simulink model "joy_stick_waypoints"  (R2024b)
settings: Solver=FixedStepAuto  StartTime=0.0  StopTime=inf  FixedStep=0.01  RelTol=1e-3
libraries: vrlib x3, aerolibutil x2
settings Model: Creator=vince  LastModifiedBy=vince

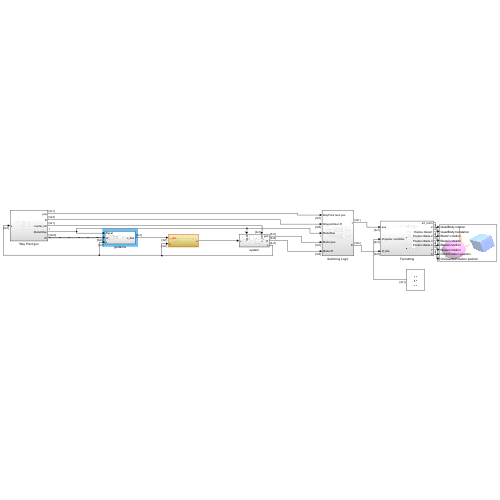
[thumbnail: Simulink's stored preview of the top-level diagram]
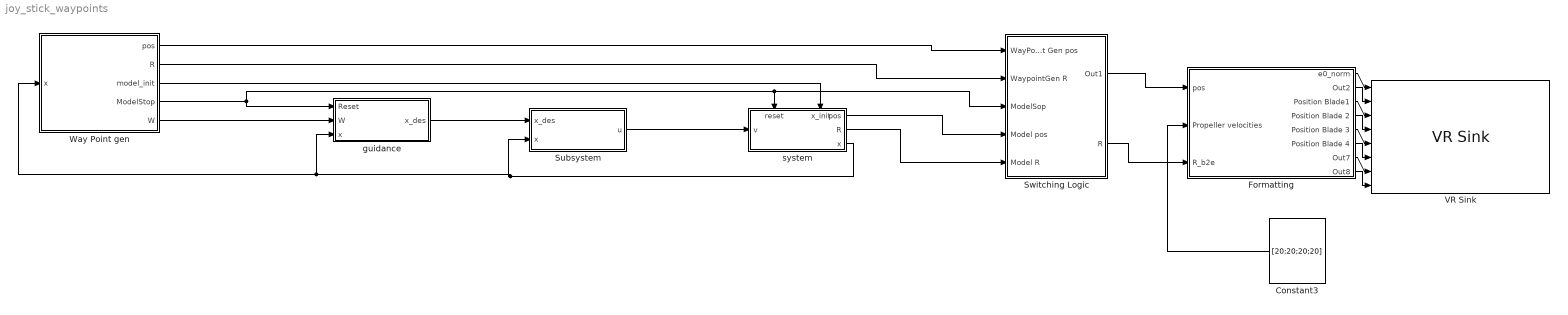
== system joy_stick_waypoints ==
  Constant3 : Constant  Value=[20;20;20;20]  VectorParams1D=off
  Formatting : Subsystem
  Subsystem : Subsystem
  Switching Logic : Subsystem
  VR Sink : vrlib/VR Sink  InstantiateOnLoad=on  SampleTime=12*0.005  ViewEnable=on  RemoteChange=off  RemoteView=off  FieldsWritten=QuadBody.rotation.4.1.1.double#QuadBody.translation.3.1.1.double#Blade1.rotation.4.1.1.double#Blade3.rotation.4.1.1.double#Blade2.rotation.4.1.1.double#Blade4.rotation.4.1.1.double#IsoNoRotation.position.3.1.1.double#OnQuadNoRotation.position.3.1.1.double  WorldFileName=Quadcopter_VR.wrl  AutoView=on  VideoDimensions=[]  AllowVariableSize=off  FigureProperties="{'Position', 'Name', 'Viewpoint', 'CameraBound', 'CameraDirection', 'CameraPosition', 'CameraUpVector', 'ZoomFactor', 'Antialiasing', 'Headlight', 'Lighting', 'Sound', 'StatusBar', 'Stereo3D', 'Stereo3DCameraOffset', 'Stereo3DHIT', 'ToolBar', 'Textures', 'Transparency', 'Triad', 'Wireframe', 'NavZones', 'NavMode', 'NavSpeed', 'CaptureFileFormat', 'CaptureFileName', 'Record2DCompressMethod', 'Record2DCompressQuality', 'Record2D', 'Record2DFileName', 'Record2DFPS', 'NavPanel'; [1.8747142857142856e+03   6.0128571428571422e+02   5.7600000000000000e+02   3.5000000000000000e+02], '', 'Chase - No Rotation', 'on', [0.0000000000000000e+00   0.0000000000000000e+00  -1.0000000000000000e+00], [0.0000000000000000e+00   0.0000000000000000e+00   0.0000000000000000e+00], [0.0000000000000000e+00   1.0000000000000000e+00   0.0000000000000000e+00], [1.0000000000000000e+00], 'on', 'on', 'on', 'on', 'on', 'off', [1.0000000149011612e-01], [0.0000000000000000e+00], 'on', 'on', 'on', 'none', 'off', 'off', 'fly', 'normal', 'tif', '%f_anim_%n.tif', 'auto', [7.5000000000000000e+01], 'off', '%f_anim_%n.avi', 'auto', 'halfbar'}"
  Way Point gen : Subsystem
  guidance : Subsystem
  system : Subsystem
      settings: PortSchema="{\"entries\":[{\"content\":{\"sides\":[{\"content\":{\"connectorIds\":[\"In1\"]},\"type\":\"ConnectorPlacement.EquallySpacedRectSide\",\"uuid\":\"24ab920f-ecdf-46b8-bd8f-9678a712bec3\"},{\"content\":{\"connectorIds\":[\"Out1\",\"Out2\",\"Out3\"],\"side\":\"RIGHT\"},\"type\":\"ConnectorPlacement.EquallySpacedRectSide\",\"uuid\":\"385c249c-ba59-490a-8b19-b03d9723e494\"},{\"content\":{\"connectorIds\":[\"In2\",\"In3\"],\"side\":\"TOP\"},\"type\":\"ConnectorPlacement.EquallySpacedRectSide\",\"uuid\":\"86d78a8a-2549-4abc-bd3a-7c80a79ae3d5\"}]},\"type\":\"ConnectorPlacement.EquallySpacedConnector\",\"uuid\":\"734c9ef5-af39-4002-a137-da897c88a198\"}],\"packageUris\":[\"http://schema.mathworks.com/mf0/Connector/R2020b\"],\"version\":\"1.0\"}"
  wires:
  Constant3/1 -> Formatting/2(Propeller velocities)
  Formatting/4(Position Blade 2) -> VR Sink/4
  Formatting/1(e0_norm) -> VR Sink/1
  Formatting/3(Position Blade1) -> VR Sink/3
  Formatting/8(Out8) -> VR Sink/8
  Formatting/7(Out7) -> VR Sink/7
  Formatting/5(Position Blade 3) -> VR Sink/5
  Formatting/6(Position Blade 4) -> VR Sink/6
  Formatting/2(Out2) -> VR Sink/2
  system/1(pos) -> Switching Logic/4(Model pos)
  Subsystem/1(u) -> system/1(v)
  guidance/1(x_des) -> Subsystem/1(x_des)
  Way Point gen/5(W) -> guidance/2(W)
  Way Point gen/3(model_init) -> system/3(x_init)
  Way Point gen/1(pos) -> Switching Logic/1(WayPoint Gen pos)
  Switching Logic/1(Out1) -> Formatting/1(pos)
  Switching Logic/2(R) -> Formatting/3(R_b2e)
  system/2(R) -> Switching Logic/5(Model R)
  system/3(x) -> Way Point gen/1(x), guidance/3(x), Subsystem/2(x)
  Way Point gen/4(ModelStop) -> system/2(reset), Switching Logic/3(ModelSop), guidance/1(Reset)
  Way Point gen/2(R) -> Switching Logic/2(WaypointGen R)

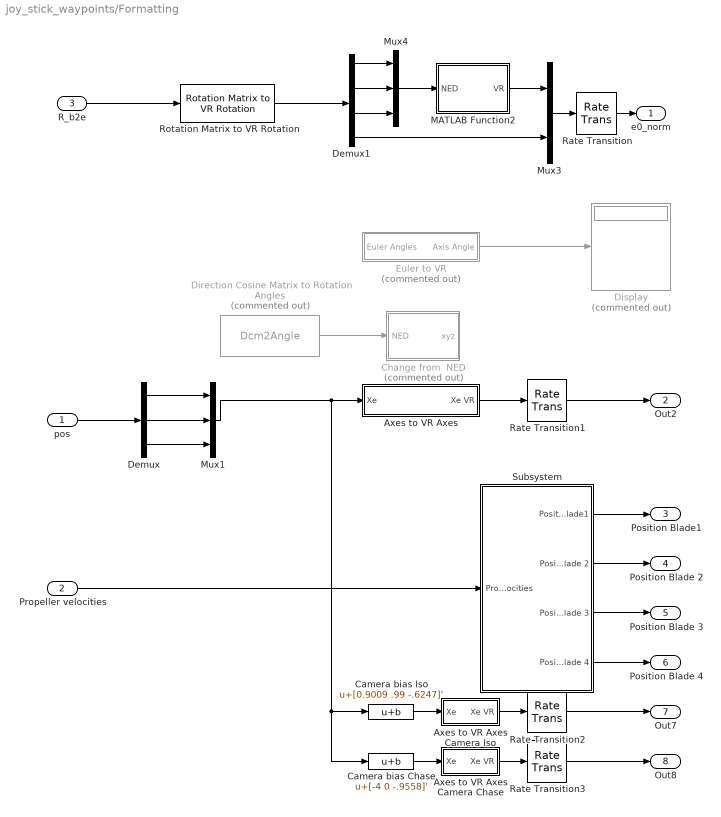
== system joy_stick_waypoints/Formatting ==
  pos : Inport
  Propeller velocities : Inport  Port=2
  R_b2e : Inport  Port=3
  Axes to VR Axes : Subsystem
  Axes to VR Axes Camera Chase : Subsystem
  Axes to VR Axes Camera Iso : Subsystem
  Camera bias Chase : Bias  Bias=[-4 0 -.9558]'  SaturateOnIntegerOverflow=off
  Camera bias Iso : Bias  Bias=[0.9009 .99 -.6247]'  SaturateOnIntegerOverflow=off
  Change from  NED : MATLAB Function  Commented=on  TreatAsAtomicUnit=on
  Demux : Demux  Outputs=3
  Demux1 : Demux
  Direction Cosine Matrix to Rotation Angles : Dcm2Angle  Commented=on
      settings: AttributesFormatString=Rotation Order: %<rotationOrder>
  Display : Display  Commented=on
  Euler to VR : Subsystem  Commented=on
  MATLAB Function2 : MATLAB Function  TreatAsAtomicUnit=on
  Mux1 : Mux  Inputs=3
  Mux3 : Mux  Inputs=2
  Mux4 : Mux  Inputs=3
  Rate Transition{,1..3} (4 alike) : RateTransition
  Rotation Matrix to VR Rotation : vrlib/Utilities/Rotation Matrix to VR Rotation  maxzero=1e-12
  Subsystem : Subsystem
  e0_norm : Outport
  Out2 : Outport  Port=2
  Position Blade1 : Outport  Port=3
  Position Blade 2 : Outport  Port=4
  Position Blade 3 : Outport  Port=5
  Position Blade 4 : Outport  Port=6
  Out7 : Outport  Port=7
  Out8 : Outport  Port=8
  wires:
  Rate Transition2/1 -> Out7/1
  Propeller velocities/1 -> Subsystem/1(Propeller velocities)
  Subsystem/3(Position Blade 3) -> Position Blade 3/1
  Subsystem/1(Position Blade1) -> Position Blade1/1
  Camera bias Chase/1 -> Axes to VR Axes Camera Chase/1(Xe)
  Axes to VR Axes Camera Chase/1(Xe VR) -> Rate Transition3/1
  Subsystem/2(Position Blade 2) -> Position Blade 2/1
  Axes to VR Axes Camera Iso/1(Xe VR) -> Rate Transition2/1
  Axes to VR Axes/1(Xe VR) -> Rate Transition1/1
  Rate Transition1/1 -> Out2/1
  Camera bias Iso/1 -> Axes to VR Axes Camera Iso/1(Xe)
  Mux1/1 -> Camera bias Chase/1, Camera bias Iso/1, Axes to VR Axes/1(Xe)
  Rate Transition3/1 -> Out8/1
  Subsystem/4(Position Blade 4) -> Position Blade 4/1
  Demux/2 -> Mux1/2
  Demux/3 -> Mux1/3
  pos/1 -> Demux/1
  Demux/1 -> Mux1/1
  Euler to VR/1(Axis Angle) -> Display/1
  Direction Cosine Matrix to Rotation Angles/1 -> Change from  NED/1(NED)
  Demux1/1 -> Mux4/1
  Demux1/2 -> Mux4/2
  MATLAB Function2/1(VR) -> Mux3/1
  R_b2e/1 -> Rotation Matrix to VR Rotation/1
  Mux4/1 -> MATLAB Function2/1(NED)
  Rotation Matrix to VR Rotation/1 -> Demux1/1
  Demux1/4 -> Mux3/2
  Demux1/3 -> Mux4/3
  Mux3/1 -> Rate Transition/1
  Rate Transition/1 -> e0_norm/1

== system joy_stick_waypoints/Subsystem ==
  x_des : Inport
  x : Inport  Port=2
  Gain : Gain  Gain=-eye(4)  Multiplication=Matrix(K*u)
  Sum : Sum  Inputs=|-+
  u : Outport
  wires:
  Gain/1 -> u/1
  Sum/1 -> Gain/1
  x/1 -> Sum/2
  x_des/1 -> Sum/1

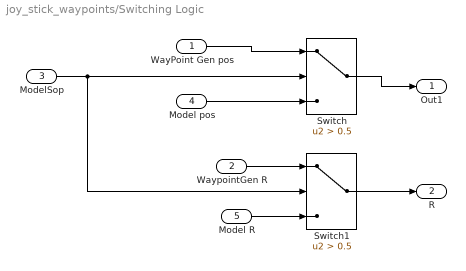
== system joy_stick_waypoints/Switching Logic ==
  WayPoint Gen pos : Inport
  WaypointGen R : Inport  Port=2
  ModelSop : Inport  Port=3
  Model pos : Inport  Port=4
  Model R : Inport  Port=5
  Switch : Switch  Criteria=u2 > Threshold  Threshold=0.5  SaturateOnIntegerOverflow=off  InputSameDT=off
  Switch1 : Switch  Criteria=u2 > Threshold  Threshold=0.5  SaturateOnIntegerOverflow=off  InputSameDT=off
  Out1 : Outport
  R : Outport  Port=2
  wires:
  Model pos/1 -> Switch/3
  ModelSop/1 -> Switch1/2, Switch/2
  WayPoint Gen pos/1 -> Switch/1
  Switch/1 -> Out1/1
  WaypointGen R/1 -> Switch1/1
  Model R/1 -> Switch1/3
  Switch1/1 -> R/1

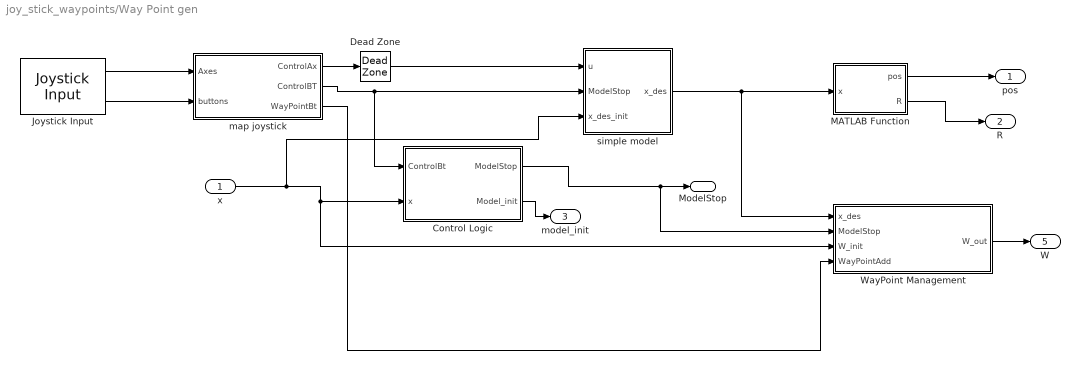
== system joy_stick_waypoints/Way Point gen ==
  x : Inport
  Control Logic : Subsystem
  Dead Zone : DeadZone  LowerValue=-0.1  UpperValue=0.1
  Joystick Input : vrlib/Joystick Input  joyid=1  adjustports=on  forcefeed=off
  MATLAB Function : MATLAB Function  TreatAsAtomicUnit=on
  WayPoint Management : MATLAB Function  TreatAsAtomicUnit=on
  map joystick : MATLAB Function  TreatAsAtomicUnit=on
  simple model : Subsystem
  pos : Outport
  R : Outport  Port=2
  model_init : Outport  Port=3
  ModelStop : Outport  Port=4
  W : Outport  Port=5
  wires:
  Joystick Input/2 -> map joystick/2(buttons)
  Joystick Input/1 -> map joystick/1(Axes)
  map joystick/1(ControlAx) -> Dead Zone/1
  Dead Zone/1 -> simple model/1(u)
  map joystick/2(ControlBT) -> Control Logic/1(ControlBt), simple model/2(ModelStop)
  x/1 -> WayPoint Management/3(W_init), Control Logic/2(x), simple model/3(x_des_init)
  simple model/1(x_des) -> MATLAB Function/1(x), WayPoint Management/1(x_des)
  map joystick/3(WayPointBt) -> WayPoint Management/4(WayPointAdd)
  WayPoint Management/1(W_out) -> W/1
  Control Logic/1(ModelStop) -> ModelStop/1, WayPoint Management/2(ModelStop)
  Control Logic/2(Model_init) -> model_init/1
  MATLAB Function/1(pos) -> pos/1
  MATLAB Function/2(R) -> R/1

== system joy_stick_waypoints/guidance ==
  Reset : Inport
  W : Inport  Port=2
  x : Inport  Port=3
  select way point : MATLAB Function  TreatAsAtomicUnit=on
  x_des : Outport
  wires:
  W/1 -> select way point/1(W)
  x/1 -> select way point/2(x)
  select way point/1(x_des) -> x_des/1
  Reset/1 -> select way point/3(reset)

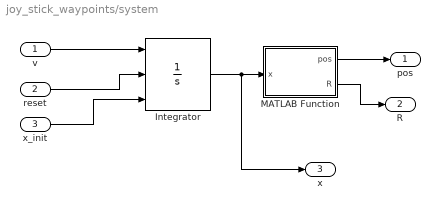
== system joy_stick_waypoints/system ==
  v : Inport
  reset : Inport  Port=2
  x_init : Inport  Port=3
  Integrator : Integrator  Priority=1  ExternalReset=level  InitialConditionSource=external
  MATLAB Function : MATLAB Function  TreatAsAtomicUnit=on
  pos : Outport
  R : Outport  Port=2
  x : Outport  Port=3
  wires:
  v/1 -> Integrator/1
  x_init/1 -> Integrator/3
  reset/1 -> Integrator/2
  MATLAB Function/1(pos) -> pos/1
  MATLAB Function/2(R) -> R/1
  Integrator/1 -> x/1, MATLAB Function/1(x)

== system joy_stick_waypoints/Formatting/Axes to VR Axes ==
  Xe : Inport
  Demux : Demux  Outputs=3
      settings: DisplayOption=none
  Mux : Mux  Inputs=3
  rad-->deg1 : Gain  Gain=-1  SaturateOnIntegerOverflow=on  OutDataTypeStr=Inherit: Same as input  ParamDataTypeStr=Inherit: Same as input
  Xe VR : Outport  VectorParamsAs1DForOutWhenUnconnected=off
  wires:
  Xe/1 -> Demux/1
  Demux/1 -> Mux/1
  Demux/3 -> rad-->deg1/1
  Mux/1 -> Xe VR/1
  rad-->deg1/1 -> Mux/2
  Demux/2 -> Mux/3

== system joy_stick_waypoints/Formatting/Axes to VR Axes Camera Chase ==
  Xe : Inport
  Demux : Demux  Outputs=3
      settings: DisplayOption=none
  Mux : Mux  Inputs=3
  rad-->deg1 : Gain  Gain=-1  SaturateOnIntegerOverflow=on  OutDataTypeStr=Inherit: Same as input  ParamDataTypeStr=Inherit: Same as input
  Xe VR : Outport  VectorParamsAs1DForOutWhenUnconnected=off
  wires:
  Xe/1 -> Demux/1
  Demux/1 -> Mux/1
  Demux/3 -> rad-->deg1/1
  Mux/1 -> Xe VR/1
  rad-->deg1/1 -> Mux/2
  Demux/2 -> Mux/3

== system joy_stick_waypoints/Formatting/Axes to VR Axes Camera Iso ==
  Xe : Inport
  Demux : Demux  Outputs=3
      settings: DisplayOption=none
  Mux : Mux  Inputs=3
  rad-->deg1 : Gain  Gain=-1  SaturateOnIntegerOverflow=on  OutDataTypeStr=Inherit: Same as input  ParamDataTypeStr=Inherit: Same as input
  Xe VR : Outport  VectorParamsAs1DForOutWhenUnconnected=off
  wires:
  Demux/2 -> Mux/3
  rad-->deg1/1 -> Mux/2
  Mux/1 -> Xe VR/1
  Demux/3 -> rad-->deg1/1
  Demux/1 -> Mux/1
  Xe/1 -> Demux/1

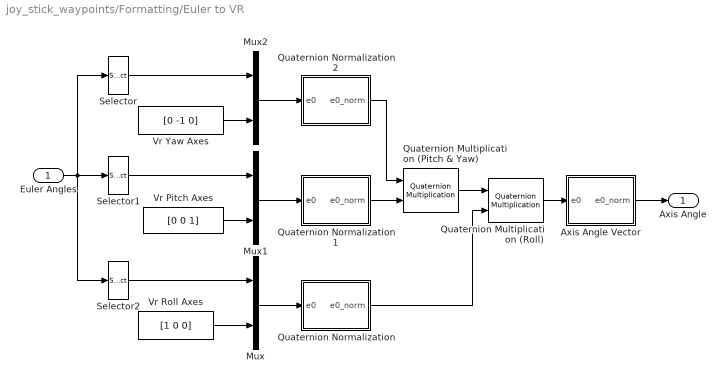
== system joy_stick_waypoints/Formatting/Euler to VR ==
  Euler Angles : Inport
  Axis Angle Vector : Subsystem
  Mux : Mux  Inputs=2
  Mux1 : Mux  Inputs=2
  Mux2 : Mux  Inputs=2
  Quaternion Multiplication (Pitch & Yaw) : aerolibutil/Quaternion Multiplication
  Quaternion Multiplication (Roll) : aerolibutil/Quaternion Multiplication
  Quaternion Normalization : Subsystem
  Quaternion Normalization1 : Subsystem
  Quaternion Normalization2 : Subsystem
  Selector : Selector  InputPortWidth=3  IndexOptions=Index vector (dialog)  Indices=[3]  OutputSizes=1
  Selector1 : Selector  InputPortWidth=3  IndexOptions=Index vector (dialog)  Indices=[2]  OutputSizes=1
  Selector2 : Selector  InputPortWidth=3  IndexOptions=Index vector (dialog)  Indices=[1]  OutputSizes=1
  Vr Pitch Axes : Constant  Value=[0 0 1]
  Vr Roll Axes : Constant  Value=[1 0 0]
  Vr Yaw Axes : Constant  Value=[0 -1 0]
  Axis Angle : Outport  VectorParamsAs1DForOutWhenUnconnected=off
  wires:
  Quaternion Multiplication (Roll)/1 -> Axis Angle Vector/1(e0)
  Axis Angle Vector/1(e0_norm) -> Axis Angle/1
  Quaternion Normalization/1(e0_norm) -> Quaternion Multiplication (Roll)/2
  Quaternion Normalization2/1(e0_norm) -> Quaternion Multiplication (Pitch & Yaw)/1
  Quaternion Normalization1/1(e0_norm) -> Quaternion Multiplication (Pitch & Yaw)/2
  Mux2/1 -> Quaternion Normalization2/1(e0)
  Mux1/1 -> Quaternion Normalization1/1(e0)
  Mux/1 -> Quaternion Normalization/1(e0)
  Selector/1 -> Mux2/1
  Vr Yaw Axes/1 -> Mux2/2
  Selector1/1 -> Mux1/1
  Vr Pitch Axes/1 -> Mux1/2
  Selector2/1 -> Mux/1
  Vr Roll Axes/1 -> Mux/2
  Euler Angles/1 -> Selector2/1, Selector1/1, Selector/1
  Quaternion Multiplication (Pitch & Yaw)/1 -> Quaternion Multiplication (Roll)/1

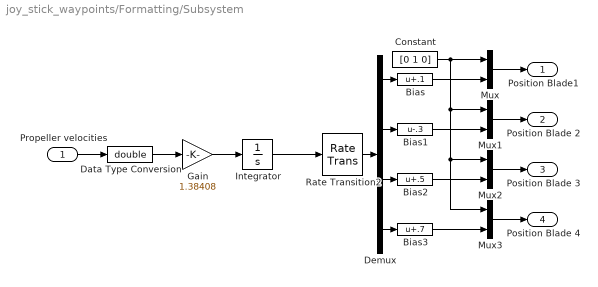
== system joy_stick_waypoints/Formatting/Subsystem ==
  Propeller velocities : Inport
  Bias : Bias  Bias=.1  SaturateOnIntegerOverflow=off
  Bias1 : Bias  Bias=-.3  SaturateOnIntegerOverflow=off
  Bias2 : Bias  Bias=.5  SaturateOnIntegerOverflow=off
  Bias3 : Bias  Bias=.7  SaturateOnIntegerOverflow=off
  Constant : Constant  Value=[0 1 0]
  Data Type Conversion : DataTypeConversion  OutDataTypeStr=double  SaturateOnIntegerOverflow=off  RndMeth=Floor
  Demux : Demux
  Gain : Gain  Gain=1.38408
  Integrator : Integrator  InitialCondition=[.1 ; .2 ;-.3 ;-.4]  WrapState=on  WrappedStateUpperValue=2*pi  WrappedStateLowerValue=-2*pi
  Mux{,1..3} (4 alike) : Mux  Inputs=2
  Rate Transition2 : RateTransition
  Position Blade1 : Outport  VectorParamsAs1DForOutWhenUnconnected=off
  Position Blade 2 : Outport  Port=2  VectorParamsAs1DForOutWhenUnconnected=off
  Position Blade 3 : Outport  Port=3  VectorParamsAs1DForOutWhenUnconnected=off
  Position Blade 4 : Outport  Port=4  VectorParamsAs1DForOutWhenUnconnected=off
  wires:
  Bias3/1 -> Mux3/2
  Mux3/1 -> Position Blade 4/1
  Bias1/1 -> Mux1/2
  Bias2/1 -> Mux2/2
  Demux/2 -> Bias1/1
  Constant/1 -> Mux3/1, Mux2/1, Mux1/1, Mux/1
  Mux1/1 -> Position Blade 2/1
  Mux2/1 -> Position Blade 3/1
  Integrator/1 -> Rate Transition2/1
  Mux/1 -> Position Blade1/1
  Demux/3 -> Bias2/1
  Bias/1 -> Mux/2
  Propeller velocities/1 -> Data Type Conversion/1
  Demux/4 -> Bias3/1
  Rate Transition2/1 -> Demux/1
  Demux/1 -> Bias/1
  Data Type Conversion/1 -> Gain/1
  Gain/1 -> Integrator/1

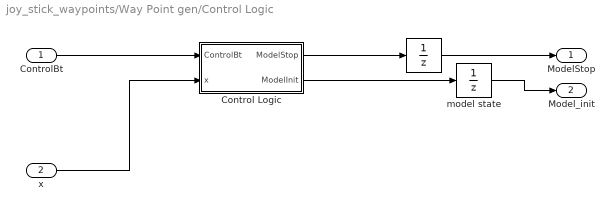
== system joy_stick_waypoints/Way Point gen/Control Logic ==
  ControlBt : Inport
  x : Inport  Port=2
  " " : UnitDelay  SampleTime=-1  HasFrameUpgradeWarning=on
  Control Logic : MATLAB Function  Priority=0  TreatAsAtomicUnit=on
  model state : UnitDelay  InitialCondition=[30;30;-10;0]  SampleTime=-1  HasFrameUpgradeWarning=on
  ModelStop : Outport
  Model_init : Outport  Port=2
  wires:
  ControlBt/1 -> Control Logic/1(ControlBt)
  x/1 -> Control Logic/2(x)
  Control Logic/1(ModelStop) -> " "/1
  " "/1 -> ModelStop/1
  Control Logic/2(ModelInit) -> model state/1
  model state/1 -> Model_init/1

== system joy_stick_waypoints/Way Point gen/simple model ==
  u : Inport
  ModelStop : Inport  Port=2
  x_des_init : Inport  Port=3
  Gain : Gain
  Integrator : Integrator  ExternalReset=rising  InitialConditionSource=external
  x_des : Outport
  wires:
  Gain/1 -> Integrator/1
  x_des_init/1 -> Integrator/3
  u/1 -> Gain/1
  ModelStop/1 -> Integrator/2
  Integrator/1 -> x_des/1

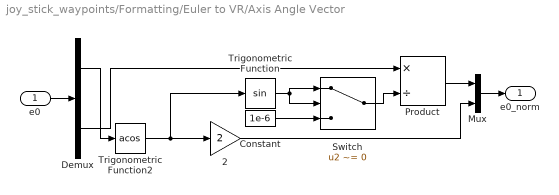
== system joy_stick_waypoints/Formatting/Euler to VR/Axis Angle Vector ==
  e0 : Inport
  2 : Gain  Gain=2  SaturateOnIntegerOverflow=on  OutDataTypeStr=Inherit: Same as input  ParamDataTypeStr=Inherit: Same as input
  Constant : Constant  Value=1e-6
  Demux : Demux  Outputs=[1 3 ]
      settings: DisplayOption=none
  Mux : Mux  Inputs=2
  Product : Product  Inputs=*/  InputSameDT=on  SaturateOnIntegerOverflow=on  OutDataTypeStr=Inherit: Same as first input
  Switch : Switch  Criteria=u2 ~= 0  SaturateOnIntegerOverflow=off  InputSameDT=off
  Trigonometric Function : Trigonometry
  Trigonometric Function2 : Trigonometry  Operator=acos
  e0_norm : Outport  VectorParamsAs1DForOutWhenUnconnected=off
  wires:
  Demux/1 -> Trigonometric Function2/1
  Demux/2 -> Product/1
  Mux/1 -> e0_norm/1
  Product/1 -> Mux/1
  2/1 -> Mux/2
  Trigonometric Function/1 -> Switch/1, Switch/2
  Trigonometric Function2/1 -> Trigonometric Function/1, 2/1
  e0/1 -> Demux/1
  Constant/1 -> Switch/3
  Switch/1 -> Product/2

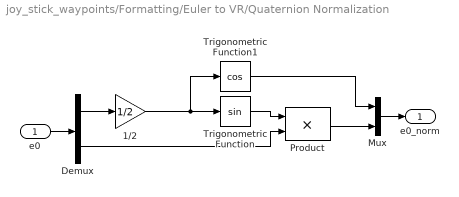
== system joy_stick_waypoints/Formatting/Euler to VR/Quaternion Normalization ==
  e0 : Inport
  1/2 : Gain  Gain=1/2  SaturateOnIntegerOverflow=on  OutDataTypeStr=Inherit: Same as input  ParamDataTypeStr=Inherit: Same as input
  Demux : Demux  Outputs=[1 3]
      settings: DisplayOption=none
  Mux : Mux  Inputs=2
  Product : Product  InputSameDT=on  SaturateOnIntegerOverflow=on  OutDataTypeStr=Inherit: Same as first input
  Trigonometric Function : Trigonometry
  Trigonometric Function1 : Trigonometry  Operator=cos
  e0_norm : Outport  VectorParamsAs1DForOutWhenUnconnected=off
  wires:
  Trigonometric Function1/1 -> Mux/1
  Demux/2 -> Product/2
  Demux/1 -> 1/2/1
  Mux/1 -> e0_norm/1
  Product/1 -> Mux/2
  Trigonometric Function/1 -> Product/1
  1/2/1 -> Trigonometric Function1/1, Trigonometric Function/1
  e0/1 -> Demux/1

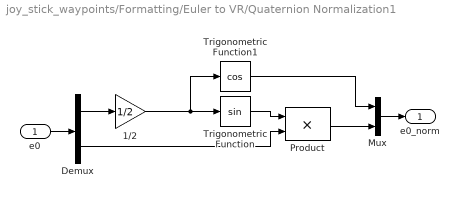
== system joy_stick_waypoints/Formatting/Euler to VR/Quaternion Normalization1 ==
  e0 : Inport
  1/2 : Gain  Gain=1/2  SaturateOnIntegerOverflow=on  OutDataTypeStr=Inherit: Same as input  ParamDataTypeStr=Inherit: Same as input
  Demux : Demux  Outputs=[1 3]
      settings: DisplayOption=none
  Mux : Mux  Inputs=2
  Product : Product  InputSameDT=on  SaturateOnIntegerOverflow=on  OutDataTypeStr=Inherit: Same as first input
  Trigonometric Function : Trigonometry
  Trigonometric Function1 : Trigonometry  Operator=cos
  e0_norm : Outport  VectorParamsAs1DForOutWhenUnconnected=off
  wires:
  e0/1 -> Demux/1
  1/2/1 -> Trigonometric Function/1, Trigonometric Function1/1
  Trigonometric Function/1 -> Product/1
  Product/1 -> Mux/2
  Mux/1 -> e0_norm/1
  Demux/1 -> 1/2/1
  Demux/2 -> Product/2
  Trigonometric Function1/1 -> Mux/1

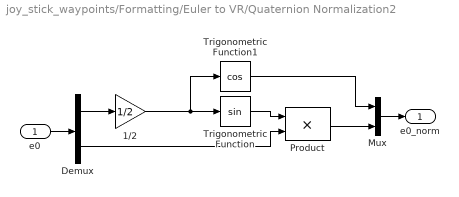
== system joy_stick_waypoints/Formatting/Euler to VR/Quaternion Normalization2 ==
  e0 : Inport
  1/2 : Gain  Gain=1/2  SaturateOnIntegerOverflow=on  OutDataTypeStr=Inherit: Same as input  ParamDataTypeStr=Inherit: Same as input
  Demux : Demux  Outputs=[1 3]
      settings: DisplayOption=none
  Mux : Mux  Inputs=2
  Product : Product  InputSameDT=on  SaturateOnIntegerOverflow=on  OutDataTypeStr=Inherit: Same as first input
  Trigonometric Function : Trigonometry
  Trigonometric Function1 : Trigonometry  Operator=cos
  e0_norm : Outport  VectorParamsAs1DForOutWhenUnconnected=off
  wires:
  Trigonometric Function1/1 -> Mux/1
  Demux/2 -> Product/2
  Demux/1 -> 1/2/1
  Mux/1 -> e0_norm/1
  Product/1 -> Mux/2
  Trigonometric Function/1 -> Product/1
  1/2/1 -> Trigonometric Function1/1, Trigonometric Function/1
  e0/1 -> Demux/1

== matlab function joy_stick_waypoints/Formatting/Change from  NED ==
  data: NED input; xyz output
function xyz = fcn(NED)
xyz=zeros([4,1]);
xyz(1)=NED(1);
xyz(2)=-NED(3);
xyz(3)=NED(2);
xyz(4)=NED(4);

== matlab function joy_stick_waypoints/guidance/select way point ==
  settings: updateMethod=DISCRETE
  data: W input size=[4,inf]; x_des output; x input size=[4,1]; reset input
function x_des = fcn(W,x,reset)

persistent i;
if isempty(i)
    i=1;
end

if reset==true
    i=1;
    x_des=zeros([4,1]);
    return;
end



thres=0.2;
if norm(W(:,i)-x)<=thres
    i=i+1;
    if i>size(W,2)
        i=size(W,2);
    end
end

x_des=zeros([4,1]);
x_des(:)=W(:,i);

== matlab function joy_stick_waypoints/Way Point gen/map joystick ==
  data: Axes input; ControlAx output; buttons input; ControlBT output; WayPointBt output
function [ControlAx,ControlBT,WayPointBt] = fcn(Axes,buttons)
%ax 3,1,2,4 bt 1,2
ControlAx=Axes([2,1,3,4]);
ControlBT=buttons(1);
WayPointBt=buttons(2);

== matlab function joy_stick_waypoints/Way Point gen/WayPoint Management ==
  settings: updateMethod=DISCRETE  sampleTime=0.01
  data: x_des input; ModelStop input; W_init input; W_out output size=[4,inf]; WayPointAdd input
function W_out = fcn(x_des, ModelStop,W_init,WayPointAdd)

persistent W;
if isempty(W)
    W=zeros([4,0]);
end

persistent WPAdd_prev;
if isempty(WPAdd_prev)
    WPAdd_prev=WayPointAdd;
end

persistent ModStop_prev
if isempty(ModStop_prev)
    ModStop_prev=ModelStop;
end

if ModelStop==true & ModStop_prev==false
    W=zeros([4,0]);
end

if WayPointAdd==true & WPAdd_prev==false
    W=[W,x_des];
end

if size(W,2)==0
    W_out=W_init;
else
    W_out=W;
end

WPAdd_prev=WayPointAdd;
ModStop_prev=ModelStop;

== matlab function joy_stick_waypoints/Way Point gen/Control Logic/Control Logic ==
  settings: updateMethod=DISCRETE  sampleTime=0.01
  data: ControlBt input; ModelStop output; x input; ModelInit output
function [ModelStop,ModelInit]  = fcn(ControlBt,x)

persistent CBT_prev;
persistent ModState;
persistent ModStop;

%initialization
if isempty(CBT_prev)
    CBT_prev=ControlBt;
    ModState=x;
    ModStop=false;
    ModelStop=false;
    ModelInit=x;
    return
end

%state update
if ControlBt==true & CBT_prev==false 
    ModStop=~ModStop;
end
if ModStop==false
    ModState=x;
end

%outputs
ModelInit=ModState;
ModelStop=ModStop;

%update internal
CBT_prev=ControlBt;

== matlab function joy_stick_waypoints/Way Point gen/MATLAB Function ==
  data: x input; pos output; R output
function [pos,R] = fcn(x)

pos=x(1:3);
yaw=x(4);

R=[cos(yaw),-sin(yaw),0;
    sin(yaw),cos(yaw),0;
    0,0,1];

== matlab function joy_stick_waypoints/system/MATLAB Function ==
  data: x input; pos output; R output
function [pos,R] = fcn(x)

pos=x(1:3);
yaw=x(4);

R=[cos(yaw),-sin(yaw),0;
    sin(yaw),cos(yaw),0;
    0,0,1];

== matlab function joy_stick_waypoints/Formatting/MATLAB Function2 ==
  data: NED input; VR output
function VR = NED2VR(NED)

x = NED(1); % north
y = NED(2); % east 
z = NED(3); % down

VR = [ -y ; -z ; x ];
